simulink model "Model"  (R2014a)
settings: Solver=ode45  StartTime=0.0  StopTime=150  RelTol=1e-3
values from neighbouring files (symbols this model uses):
  K_psi = -100    [script.m]
  psi_d = temp.ans(2,:)    [script.m]
  X = temp.ans(3,:)    [script.m]
settings Model: Creator=shivjr  LastModifiedBy=shivjr

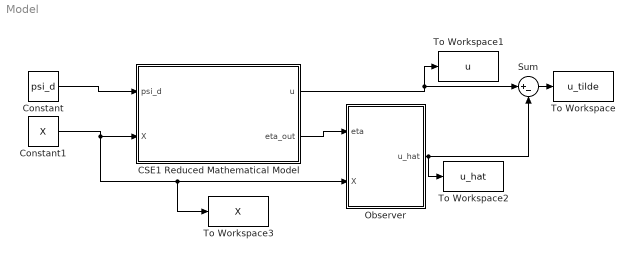
== system Model ==
  CSE1 Reduced Mathematical Model : Subsystem
  Constant : Constant  Value=psi_d
  Constant1 : Constant  Value=X
  Observer : Subsystem
  Sum : Sum  Inputs=|+-
  To Workspace : ToWorkspace  VariableName=u_tilde  SaveFormat=Timeseries  SampleTime=-1
  To Workspace1 : ToWorkspace  VariableName=u  SaveFormat=Timeseries  SampleTime=-1
  To Workspace2 : ToWorkspace  VariableName=u_hat  SaveFormat=Timeseries  SampleTime=-1
  To Workspace3 : ToWorkspace  VariableName=X  SaveFormat=Timeseries  SampleTime=-1
  wires:
  Constant/1 -> CSE1 Reduced Mathematical Model/1(psi_d)
  CSE1 Reduced Mathematical Model/1(u) -> To Workspace1/1, Sum/1
  Constant1/1 -> To Workspace3/1, Observer/2(X), CSE1 Reduced Mathematical Model/2(X)
  CSE1 Reduced Mathematical Model/2(eta_out) -> Observer/1(eta)
  Observer/1(u_hat) -> Sum/2, To Workspace2/1
  Sum/1 -> To Workspace/1

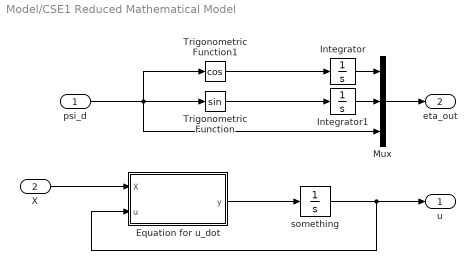
== system Model/CSE1 Reduced Mathematical Model ==
  psi_d : Inport
  X : Inport  Port=2
  Equation for u_dot : MATLAB Function  TreatAsAtomicUnit=on
  Integrator : Integrator
  Integrator1 : Integrator
  Mux : Mux  Inputs=3
  Trigonometric Function : Trigonometry
  Trigonometric Function1 : Trigonometry  Operator=cos
  something : Integrator
  u : Outport
  eta_out : Outport  Port=2
  wires:
  Mux/1 -> eta_out/1
  Integrator1/1 -> Mux/2
  Trigonometric Function/1 -> Integrator1/1
  Integrator/1 -> Mux/1
  Trigonometric Function1/1 -> Integrator/1
  psi_d/1 -> Trigonometric Function1/1, Mux/3, Trigonometric Function/1
  Equation for u_dot/1(y) -> something/1
  X/1 -> Equation for u_dot/1(X)
  something/1 -> Equation for u_dot/2(u), u/1

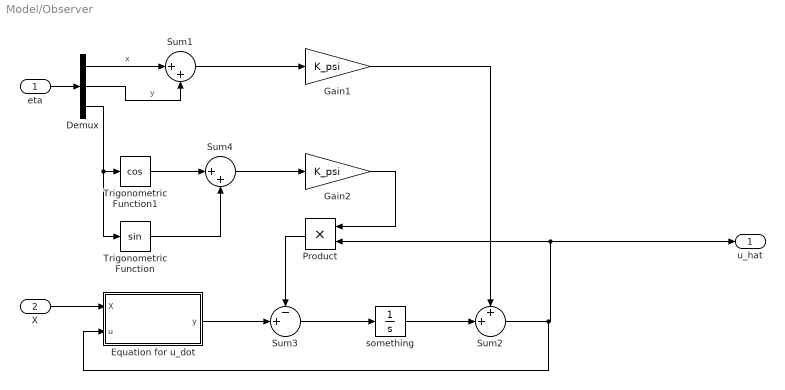
== system Model/Observer ==
  eta : Inport
  X : Inport  Port=2
  Demux : Demux  Outputs=3
  Equation for u_dot : MATLAB Function  TreatAsAtomicUnit=on
  Gain1 : Gain  Gain=K_psi
  Gain2 : Gain  Gain=K_psi
  Product : Product
  Sum1 : Sum  Inputs=|++
  Sum2 : Sum  Inputs=++|
  Sum3 : Sum  Inputs=-+|
  Sum4 : Sum  Inputs=|++
  Trigonometric Function : Trigonometry
  Trigonometric Function1 : Trigonometry  Operator=cos
  something : Integrator
  u_hat : Outport
  wires:
  something/1 -> Sum2/2
  eta/1 -> Demux/1
  Sum1/1 -> Gain1/1
  Gain1/1 -> Sum2/1
  Trigonometric Function1/1 -> Sum4/1
  Trigonometric Function/1 -> Sum4/2
  Sum4/1 -> Gain2/1
  Gain2/1 -> Product/1
  Sum3/1 -> something/1
  Product/1 -> Sum3/1
  Demux/1 -> Sum1/1  "x"
  Demux/2 -> Sum1/2  "y"
  Demux/3 -> Trigonometric Function/1, Trigonometric Function1/1
  X/1 -> Equation for u_dot/1(X)
  Equation for u_dot/1(y) -> Sum3/2
  Sum2/1 -> Equation for u_dot/2(u), Product/2, u_hat/1

== matlab function Model/Observer/Equation for u_dot ==
  data: X input; u input; y output
function y = fcn(X,u)
Xu = -0.6555;
Xuu = 0.3545;
Xuuu = -3.787;

m = 15.79;
Xu_dot = -2;
m11 = m+Xu_dot;
y = (X-(-Xu*u - Xuu*u^2 - Xuuu*u^3))/(m11);

== matlab function Model/CSE1 Reduced Mathematical Model/Equation for u_dot ==
  data: X input; u input; y output
function y = fcn(X,u)
Xu = -0.6555;
Xuu = 0.3545;
Xuuu = -3.787;

m = 15.79;
Xu_dot = -2;
m11 = m+Xu_dot;
y = (X-(-Xu*u - Xuu*u^2 - Xuuu*u^3))/(m11);
